simulink library "gyroSensorHW_sl"  (R2024b)
settings: Solver=VariableStepAuto  StartTime=0.0  StopTime=10.0  RelTol=1e-3
undefined symbols (not defined in the file): dtSim, gyroBias, gyroErrorFlag, gyroNoisePower
libraries: simulink x1
settings Model: Creator=gilbu
settings RTWCC: GPUComputeCapability=3.5

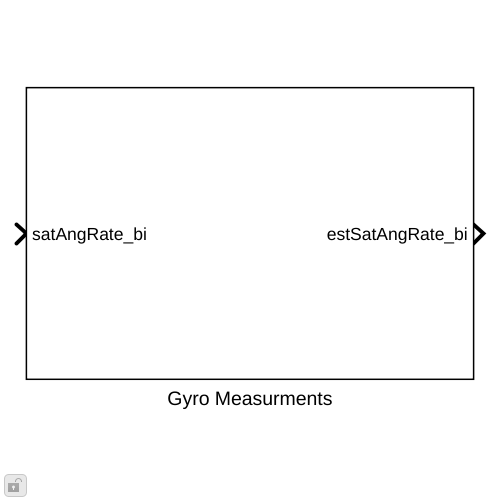
[thumbnail: Simulink's stored preview of the top-level diagram]
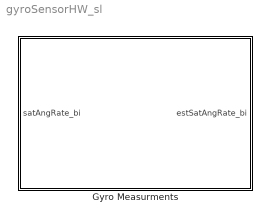
== system gyroSensorHW_sl ==
  Gyro Measurments : Subsystem  mask{gyroErrorFlag=gyroErrorFlag, gyroBias=gyroBias, gyroNoisePower=gyroNoisePower}
      mask prompts: gyroErrorFlag "Gyro Error Flag <1> [-]"; gyroBias "Gyro Bias measurment error <3> [rad/s]"; gyroNoisePower "White Noise power <1> [rad2/s3]"
      mask DialogControl DescTextVar Prompt: Simulated gyro HW for angular rate measurements. Error includes bias and White-noise. Errors can be tured on an off using gyroErrorFlag and parameters.
      mask DialogControl Control2 Prompt: Gyro Error Flag equal to one will allow guassian white noise into the angular rate measurements

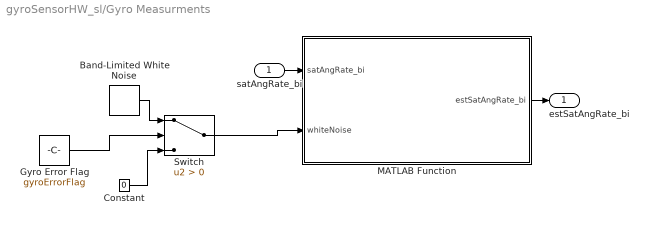
== system gyroSensorHW_sl/Gyro Measurments ==
  satAngRate_bi : Inport
  Band-Limited White Noise : simulink/Sources/Band-Limited White Noise  Cov=[gyroNoisePower]  Ts=dtSim  seed=[23341]
  Constant : Constant  Value=0
  Gyro Error Flag : Constant  Value=gyroErrorFlag
  MATLAB Function : MATLAB Function  TreatAsAtomicUnit=on
  Switch : Switch  Criteria=u2 > Threshold  SaturateOnIntegerOverflow=off  InputSameDT=off
  estSatAngRate_bi : Outport
  wires:
  Switch/1 -> MATLAB Function/2(whiteNoise)
  satAngRate_bi/1 -> MATLAB Function/1(satAngRate_bi)
  Gyro Error Flag/1 -> Switch/2
  MATLAB Function/1(estSatAngRate_bi) -> estSatAngRate_bi/1
  Band-Limited White Noise/1 -> Switch/1
  Constant/1 -> Switch/3

== matlab function gyroSensorHW_sl/Gyro Measurments/MATLAB Function ==
  data: satAngRate_bi input double size=3; estSatAngRate_bi output size=3; whiteNoise input size=1; gyroBias parameter size=3
% Author: Antonio Gil Buitrago
function estSatAngRate_bi = gyroMeasurement( ...
    satAngRate_bi,whiteNoise,... %inputs
    gyroBias...
    )
%-------------------------------------------------------------------------------
% Simulated Noise Measurement

estSatAngRate_bi = satAngRate_bi + gyroBias + whiteNoise.*ones(3,1);


%-------------------------------------------------------------------------------
end
